simulink subsystem "SolarTrack"  (R2023b)
settings: Solver=VariableStepAuto  StartTime=0.0  StopTime=10.0  RelTol=1e-3
settings Model: Creator=mrrom  LastModifiedBy=mrrom

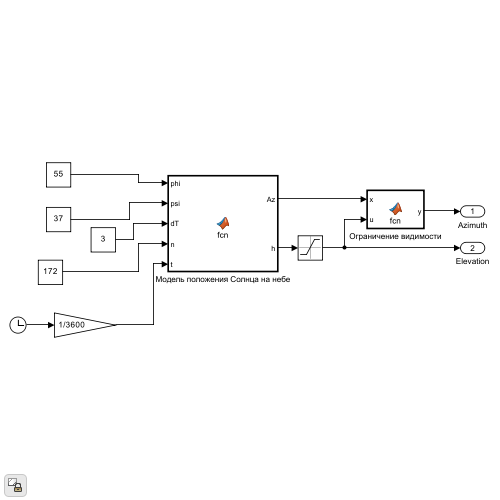
[thumbnail: Simulink's stored preview of the top-level diagram]
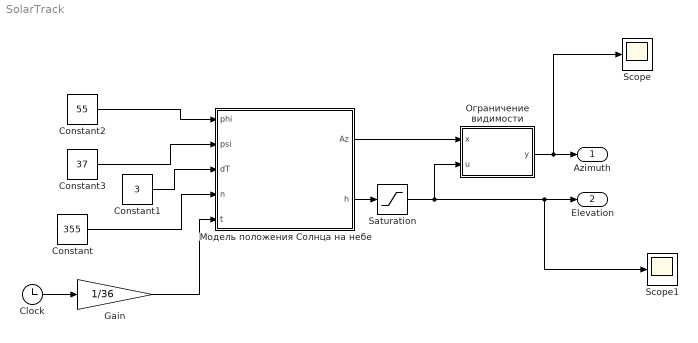
== system SolarTrack ==
  Clock : Clock
  Constant : Constant  Value=355
  Constant1 : Constant  Value=3
  Constant2 : Constant  Value=55
  Constant3 : Constant  Value=37
  Gain : Gain  Gain=1/36
  Saturation : Saturate  UpperLimit=90  LowerLimit=0
  Scope : Scope
  Scope1 : Scope
  Модель положения Солнца на небе : MATLAB Function  TreatAsAtomicUnit=on
  Ограничение видимости : MATLAB Function  TreatAsAtomicUnit=on
  Azimuth : Outport
  Elevation : Outport  Port=2
  wires:
  Модель положения Солнца на небе/2(h) -> Saturation/1
  Constant/1 -> Модель положения Солнца на небе/4(n)
  Clock/1 -> Gain/1
  Constant2/1 -> Модель положения Солнца на небе/1(phi)
  Constant3/1 -> Модель положения Солнца на небе/2(psi)
  Constant1/1 -> Модель положения Солнца на небе/3(dT)
  Ограничение видимости/1(y) -> Azimuth/1, Scope/1
  Модель положения Солнца на небе/1(Az) -> Ограничение видимости/1(x)
  Gain/1 -> Модель положения Солнца на небе/5(t)
  Saturation/1 -> Ограничение видимости/2(u), Elevation/1, Scope1/1

== matlab function SolarTrack/Модель положения Солнца на небе ==
  data: phi input; Az output; psi input; dT input; n input; h output; t input
function [Az , h]= fcn(phi,psi,dT,n,t)
% A = sin(phi)*cos(beta)
% B = cos(phi)*sin(beta)*cos(gamma)
% C = sin(beta)*sin(gamma)
% D = cos(phi)*cos(beta)
% E = sin(phi)*sin(beta)*cos(gamma)
% cos(teta) = (A-B)*sin(delta) + (C*sin(omega)+(D+E)*cos(omega))*cos(delta)
b0 = 360/365;
b = b0*(n-81);
delta = 23.45*sind(b0*(n+284));
Tuv = 1/60*(9.87*sind(2*b)-7.53*cosd(b)-1.5*sind(b));
omega = 15*(t - 12 - Tuv - dT) + psi;
tetaz = acosd(sind(phi)*sind(delta)+cosd(phi)*cosd(delta)*cosd(omega));
h = 90-tetaz;
Az =acosd((cosd(tetaz)*sind(phi)-sind(delta))/(sind(tetaz)*cosd(phi)) ...
    )*sign(omega);

== matlab function SolarTrack/Ограничение видимости ==
  data: x input; u input; y output
function y = fcn(x,u)
if u == 0
    y = 0;
else
    y = x;
end
